simulink model "MQTT"  (R2018b)
settings: Solver=VariableStepAuto  StartTime=0.0  StopTime=10.0  RelTol=1e-3
settings Model: Creator=lenovo  LastModifiedBy=lenovo

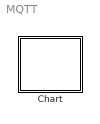
== system MQTT ==
  Chart : Stateflow chart  TreatAsAtomicUnit=on

== stateflow chart MQTT/Chart ==
